simulink subsystem "PvtSubSys_VSM_ALL"  (R2020b)
settings: Solver=VariableStepAuto  StartTime=0.0  StopTime=10.0  RelTol=1e-3
values from neighbouring files (symbols this model uses):
  P_VSM_NOH_Act_Req = 0    [VSM_All.sldd]
  P_VSM_NOH_Swt_Req = 0    [VSM_All.sldd]
undefined symbols (not defined in the file or in its folder): ACC_STATE, HWA_STATE, LCK_STATE, P_VSM_ACCSOS_SW, P_VSM_AESSwtReq, P_VSM_CruiseFunUserInputMappingWays, P_VSM_ELKSwtReq, P_VSM_ESS_VehSwtReq, P_VSM_HWA_DMS_Enable, P_VSM_ICA_HandsOffSwtReq, P_VSM_IntelligentEvaSwtReq, P_VSM_ISLSwtReq, P_VSM_LCKSwtReq, P_VSM_LDWSwtReq, P_VSM_LKASwtReq, P_VSM_LSSSwtReq, P_VSM_PowerTrainConfig, P_VSM_SOSContinueTime, P_VSM_SOSSpdLimit, P_VSM_TSR_Dis_keep_SPL_Table, P_VSM_TSR_Dis_keep_SPLend, P_VSM_TSR_Dis_keep_TS_Table, P_VSM_TSR_Ena_SPLSupp_Table, P_VSM_TSR_Ena_TS_Table, P_VSM_TSR_SLIF_Speed_High, P_VSM_TSR_SLIF_Speed_Low, P_VSM_TSR_SLW_SnvtySwitch, P_VSM_TSR_SLW_Speed_Delta_disable, P_VSM_TSR_SLW_Speed_Delta_enable, P_VSM_TSR_SLW_Speed_High, P_VSM_TSR_SLW_Speed_Low, P_VSM_TSR_SLW_TrafEyeAvtiveDist, P_VSM_TSR_SLW_Warning_Time, P_VSM_TSR_SteerWheelAngle, P_VSM_TSR_SWS_speed_withDir, P_VSM_TSR_SWS_speed_woDir, P_VSM_TSRSwtReq, P_VSM_TSRWarnSwtReq, TJA_STATE, User_LC_ALCswt, User_LC_DrvConfirm, User_LC_DrvLCswt, User_LC_DrvOverride, User_LC_LeTurnNextLineReq, User_LC_RiTurnNextLineReq, User_LC_TurnMostLeLineReq, User_LC_TurnMostRiLineReq, User_LeTurnLmpOn, User_RiTurnLmpOn
libraries: simulink x51
(part 5 of 7)

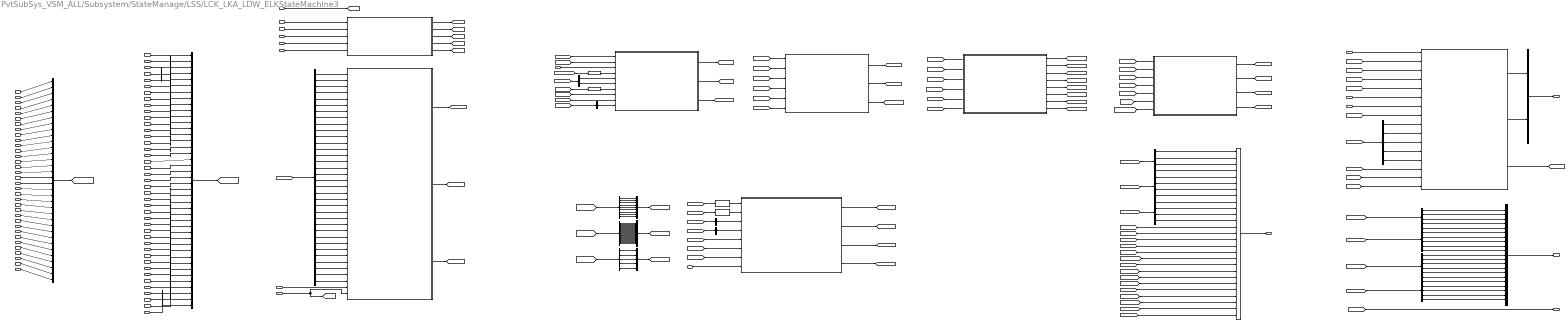
== system PvtSubSys_VSM_ALL/Subsystem/StateManage/LSS/LCK_LKA_LDW_ELKStateMachine3 ==
  VehConfig : Inport
  IFC_FailSafe : Inport  Port=2
  LCKError : Inport  Port=3
  LKAError : Inport  Port=4
  LDWError : Inport  Port=5
  ELKError : Inport  Port=6
  LCKLane_A0 : Inport  Port=7
  LCKLane_A1 : Inport  Port=8
  LCKLane_A2 : Inport  Port=9
  LCKLane_A3 : Inport  Port=10
  LCKLane_Valid : Inport  Port=11
  laneLeftA0 : Inport  Port=12
  laneLeftA1 : Inport  Port=13
  laneLeftA2 : Inport  Port=14
  laneLeftA3 : Inport  Port=15
  laneLeftValid : Inport  Port=16
  laneLeftRange : Inport  Port=17
  laneLeftType : Inport  Port=18
  laneRightA0 : Inport  Port=19
  laneRightA1 : Inport  Port=20
  laneRightA2 : Inport  Port=21
  laneRightA3 : Inport  Port=22
  laneRightValid : Inport  Port=23
  laneRightRange : Inport  Port=24
  laneRightType : Inport  Port=25
  F_LBbIsLineExist : Inport  Port=26
  F_LBdC0V : Inport  Port=27
  F_LBdC1V : Inport  Port=28
  F_LBdC2V : Inport  Port=29
  F_LBdC3V : Inport  Port=30
  RELeft_Range : Inport  Port=31
  F_RBbIsLineExist : Inport  Port=32
  F_RBdC0V : Inport  Port=33
  F_RBdC1V : Inport  Port=34
  F_RBdC2V : Inport  Port=35
  F_RBdC3V : Inport  Port=36
  RERight_Range : Inport  Port=37
  EVI_VehicleSpd_ms : Inport  Port=38
  EVI_Kap : Inport  Port=39
  EVI_alpSideSlipAngle : Inport  Port=40
  LCKIEBus : Inport  Port=41
  ELK_ObjBus : Inport  Port=42
  LIneEdgeUpdate : Inport  Port=43
  TrqK1 : Inport  Port=44
  targetExistP0 : Inport  Port=45
  HWALineValid : Inport  Port=46
  TJALineValid : Inport  Port=47
  LCKLineValid : Inport  Port=48
  HWAActive : Inport  Port=49
  TJASts : Inport  Port=50
  TJAOn : Inport  Port=51
  HWASts : Inport  Port=52
  canABSVehicleSpd : Inport  Port=53
  canABMVehDynYawRate : Inport  Port=54
  canESPVDCActive : Inport  Port=55
  canESPPTCActive : Inport  Port=56
  canESPBTCActive : Inport  Port=57
  canABSABSActive : Inport  Port=58
  HandsOffDetect : Inport  Port=59
  canSASSteerWheelAngle : Inport  Port=60
  canEPS_DriverInputTrqValue : Inport  Port=61
  canSASSteerWheelSpd : Inport  Port=62
  canABMLateralAcce : Inport  Port=63
  LongitudeAcc : Inport  Port=64
  canESP_MasterCylindBrakePress : Inport  Port=65
  canECMAccrPedlPosnDiagc : Inport  Port=66
  canEPS_LKATrqOvlDlvdSts : Inport  Port=67
  CURRENT_GEAR : Inport  Port=68
  canBCMLeftTurnSWSts : Inport  Port=69
  canBCMRightTurnSWSts : Inport  Port=70
  HandsOffWarnLevel : Inport  Port=71
  canBCMWiperSwitchSts : Inport  Port=72
  canBCMHighBeamSts : Inport  Port=73
  canBCMLowBeamSts : Inport  Port=74
  canBCMRearFogLmpSts : Inport  Port=75
  canBCMFrontFogLmpSts : Inport  Port=76
  canHUTLCKSwtReq : Inport  Port=77
  canHUTLKASwtReq : Inport  Port=78
  canHUTELKSwtReq : Inport  Port=79
  canHUTLDWSwtReq : Inport  Port=80
  IntelligentEvaSwtReq : Inport  Port=81
  IFC_SnvtySet : Inport  Port=82
  LSSSwtReq : Inport  Port=83
  ESSSts : Inport  Port=84
  PilotSts : Inport  Port=85
  BrkPedalSts : Inport  Port=86
  Bus Creator : BusCreator  Inputs=34
  Bus Creator1 : BusCreator  Inputs=27
  Bus Creator2 : BusCreator  Inputs=42
  Bus Creator3 : BusCreator  Inputs=9
  Bus Creator4 : BusCreator  Inputs=23
  Bus Creator5 : BusCreator  Inputs=5
  Bus Creator6 : BusCreator  Inputs=21
  Bus Selector : BusSelector  OutputSignals=LDW_Idle2Ready,LDW_Ready2Active,LDW_Active2Ready,LDW_Other2Idle
  Bus Selector11 : BusSelector  OutputSignals=Left_Valid,Right_Valid,Left_A0,Right_A0,C_Lanewidth
  Bus Selector12 : BusSelector  OutputSignals=LCKLane_A0,LCKLane_A1,LCKLane_A2,LCKLane_A3,LCKLane_Valid,laneLeftA0,laneLeftA1,laneLeftA2,laneLeftA3,laneLeftValid,laneLeftRange,laneLeftType,laneRightA0,laneRightA1,laneRightA2,laneRightA3,laneRightValid,laneRightRange,laneRightType,F_LBbIsLineExist,F_LBdC0V,F_LBdC1V,F_LBdC2V,F_LBdC3V,RELeft_Range,F_RBbIsLineExist,F_RBdC0V,F_RBdC1V,F_RBdC2V,F_RBdC3V,RERight_Range,EVI_VehicleSpd_ms,EVI_Kap,EVI_alpSideSlipAngle
  Bus Selector13 : BusSelector  OutputSignals=FLWhelDy,FRWhelDy
  Bus Selector14 : BusSelector  OutputSignals=Left_A0,Left_A1,Left_A2,Left_A3,Left_Valid,Right_A0,Right_A1,Right_A2,Right_A3,Right_Valid,LeftRE_A0,LeftRE_A1,LeftRE_A2,LeftRE_A3,LeftRE_Valid,RightRE_A0,RightRE_A1,RightRE_A2,RightRE_A3,RightRE_Valid,LaneCurve,LeftChange,RightChange
  Bus Selector15 : BusSelector  OutputSignals=LCK_Con_SteerAngleSpd_ LCKExit,LCK_Con_BrakePress_ LCKExit,LCK_Con_OverRide_ LCKExit,LCK_Con_AccPedalRate_LCKExit,LCK_Con_SteerWheelAngle_ LCKExit,LCK_Con_DriverInput_ LCKExit
  Bus Selector16 : BusSelector  OutputSignals=LKA_Con_SteerWheelAngle_ LKAExit,LKA_Con_DriverInput_ LKAExit,LKA_Con_SteerWheelSpd_ LKAExit,LKA_Con_BrakePressure_ LKAExit,LKA_Con_AccPedalRate_LKAExit,LKA_Con_OverRide_ LKAExit
  Bus Selector17 : BusSelector  OutputSignals=LDW_Con_AccPedalRate_LDWExit,LDW_Con_BrakePressure_ LDWExit,LDW_Con_SteerWheelSpd_ LDWExit,LDW_Con_SteerWheelAngle_ LDWExit,LDW_Con_DriverInput_ LDWExit
  Bus Selector2 : BusSelector  OutputSignals=VehConfigELK
  Bus Selector3 : BusSelector  OutputSignals=VehConfigLCKIE
  Bus Selector4 : BusSelector  OutputSignals=LKA_Idle2Ready,LKA_Ready2Active,LKA_Active2Ready,LKA_Other2Idle
  Bus Selector5 : BusSelector  OutputSignals=LCKLane_A0,LCKLane_A1,LCKLane_A2,LCKLane_A3,LCKLane_Valid
  Bus Selector6 : BusSelector  OutputSignals=IntelligentEvaSwtReq,canABSVehicleSpd,canBCMWiperSwitchSts,canBCMHighBeamSts,canBCMLowBeamSts,canBCMRearFogLmpSts,canBCMFrontFogLmpSts,canEPS_DriverInputTrqValue,HWASts
  Bus Selector7 : BusSelector  OutputSignals=EVI_VehicleSpd_ms
  Bus Selector8 : BusSelector  OutputSignals=VSM_ELK_Idle2Ready,VSM_ELK_Ready2Active,VSM_ELK_Active2Ready,VSM_ELK_Other2Idle
  Bus Selector9 : BusSelector  OutputSignals=ELK_Con_AccPedalRate_ELKExit,ELK_Con_BrakePressure_ ELKExit,ELK_Con_SteerWheelAngle_ ELKExit,ELK_Con_SteerWheelSpd_ ELKExit
  Bus Creator22 : BusCreator  Inputs=2
  Data Type Conversion : DataTypeConversion  OutDataTypeStr=boolean
  Data Type Conversion1 : DataTypeConversion  OutDataTypeStr=uint8
  Data Type Conversion2 : DataTypeConversion  OutDataTypeStr=boolean
  Data Type Conversion3 : DataTypeConversion  OutDataTypeStr=uint8
  ELKState_Machine : Subsystem
  Error : Subsystem
  HandsOffWarnLevel1 : InportShadow  Port=71
  LCK : Subsystem
  LCKIE : Subsystem  ReferencedSubsystem=PvtSubSys_VSM_LCKIE
  LDW : Subsystem
  LKA : Subsystem
  LSSHMI : Subsystem
  Signal_calculate : Subsystem  ReferencedSubsystem=PvtSubSys_VSM_SCM
  TJASts1 : InportShadow  Port=50
  canHUTLCKSwtReq1 : InportShadow  Port=77
  LCS_OutPut : Outport
  IFC_Signal : Outport  Port=2
  LSS_DATA : Outport  Port=3
  LaneARe_SP : Outport  Port=4
  wires:
  BrkPedalSts/1 -> Bus Creator2/42
  Bus Selector14/23 -> Bus Creator4/23  "<RightChange>"
  Bus Selector14/22 -> Bus Creator4/22  "<LeftChange>"
  [LANE] -> LCK/7(Lane)
  [PiloSts] -> LCK/6(PiloSts)
  PilotSts/1 -> Signal_calculate/36, [PiloSts]
  [TJA_LCKState] -> Bus Creator1/27  "TJA_LCKState"
  LCK/4(TJA_LCKState) -> [TJA_LCKState]
  [LaneARe_SP] -> LaneARe_SP/1
  Data Type Conversion3/1 -> ELKState_Machine/4(LKAState)
  Bus Creator6/1 -> LSS_DATA/1
  Bus Selector17/5 -> Bus Creator6/21  "<LDW_Con_DriverInput_ LDWExit>"
  Bus Selector17/4 -> Bus Creator6/20  "<LDW_Con_SteerWheelAngle_ LDWExit>"
  Bus Selector17/3 -> Bus Creator6/19  "<LDW_Con_SteerWheelSpd_ LDWExit>"
  Bus Selector17/2 -> Bus Creator6/18  "<LDW_Con_BrakePressure_ LDWExit>"
  Bus Selector17/1 -> Bus Creator6/17  "<LDW_Con_AccPedalRate_LDWExit>"
  Bus Selector16/6 -> Bus Creator6/16  "<LKA_Con_OverRide_ LKAExit>"
  Bus Selector15/1 -> Bus Creator6/5  "<LCK_Con_SteerAngleSpd_ LCKExit>"
  Bus Selector16/5 -> Bus Creator6/15  "<LKA_Con_AccPedalRate_LKAExit>"
  Bus Selector15/2 -> Bus Creator6/6  "<LCK_Con_BrakePress_ LCKExit>"
  Bus Selector16/4 -> Bus Creator6/14  "<LKA_Con_BrakePressure_ LKAExit>"
  Bus Selector15/3 -> Bus Creator6/7  "<LCK_Con_OverRide_ LCKExit>"
  Bus Selector9/4 -> Bus Creator6/4  "<ELK_Con_SteerWheelSpd_ ELKExit>"
  Bus Selector16/3 -> Bus Creator6/13  "<LKA_Con_SteerWheelSpd_ LKAExit>"
  Bus Selector16/1 -> Bus Creator6/11  "<LKA_Con_SteerWheelAngle_ LKAExit>"
  Bus Selector15/6 -> Bus Creator6/10  "<LCK_Con_DriverInput_ LCKExit>"
  Bus Selector15/4 -> Bus Creator6/8  "<LCK_Con_AccPedalRate_LCKExit>"
  Bus Selector9/3 -> Bus Creator6/3  "<ELK_Con_SteerWheelAngle_ ELKExit>"
  Bus Selector9/1 -> Bus Creator6/1  "<ELK_Con_AccPedalRate_ELKExit>"
  Bus Selector16/2 -> Bus Creator6/12  "<LKA_Con_DriverInput_ LKAExit>"
  Bus Selector15/5 -> Bus Creator6/9  "<LCK_Con_SteerWheelAngle_ LCKExit>"
  Bus Selector9/2 -> Bus Creator6/2  "<ELK_Con_BrakePressure_ ELKExit>"
  [LDW_Data] -> Bus Selector17/1
  [LKA_Data] -> Bus Selector16/1
  [LCK_Data] -> Bus Selector15/1
  [ELKCondition] -> Bus Selector9/1
  LSSHMI/3(Warn) -> [LKAWarning]
  LSSHMI/2(LaneAvaliability) -> Bus Creator22/2
  LSSHMI/1(Signal_HandsOffWarn) -> Bus Creator22/1
  TJASts1/1 -> LSSHMI/7(TJASts)  "TJASts"
  HandsOffWarnLevel1/1 -> LSSHMI/6(HandsOffWarnLevel)  "HandsOffWarnLevel"
  [LCK_State] -> LSSHMI/8(In8)
  [LKA_State] -> LSSHMI/5(In5)
  [ELK_State] -> LSSHMI/4(In4)
  [ELKWarn] -> LSSHMI/16(ELK_Warn)
  [LKA_Warn] -> LSSHMI/15(In15)
  [LCK_Warn] -> LSSHMI/14(LCK_Warn)
  Bus Selector11/5 -> LSSHMI/13(LaneWidth)  "<C_Lanewidth>"
  Bus Selector11/4 -> LSSHMI/12(RightA0)  "<Right_A0>"
  Bus Selector11/3 -> LSSHMI/11(LeftA0)  "<Left_A0>"
  Bus Selector11/1 -> LSSHMI/9(LeftValid)  "<Left_Valid>"
  Bus Selector11/2 -> LSSHMI/10(RightValid)  "<Right_Valid>"
  [LDW_State] -> LSSHMI/3(In3)
  [LCK_State] -> LSSHMI/2(In2)
  canHUTLCKSwtReq1/1 -> LSSHMI/1(canHUTLCKSwtReq)  "canHUTLCKSwtReq"
  [VSM_LCKIE_out] -> Bus Creator1/26
  [VSM_LCKIE_IN] -> Bus Creator1/25
  LCKIE/4 -> [VSM_LCKIE_out]
  LCKIE/3 -> [VSM_LCKIE_IN]
  Bus Selector13/2 -> ELKState_Machine/6(FRWhelDy)  "<FRWhelDy>"
  Bus Selector13/1 -> ELKState_Machine/5(FLWhelDy)  "<FLWhelDy>"
  [LKA_LDW_Signal] -> Bus Selector13/1
  [ADmix] -> LDW/5(ADmix)
  [VehConfig] -> LKA/4(VehConfig)
  [LaneARe_SP] -> LDW/4(LaneARe_SP)
  [VehConfig] -> LDW/1(VehConfig)
  LCK/2(LCK_Warn) -> [LCK_Warn]
  [LDW_Error] -> LDW/2(LDW_Error)
  LKA/2(LKA_State) -> [LKA_State]
  [LKA_LDW_Signal] -> LDW/3(LKA_LDW_Signal)
  LKA/8(LKACondition) -> [LKACondition]
  [LKA_LDW_Signal] -> LKA/2(LKA_LDW_Signal)
  LDW/1(LDW_State) -> [LDW_State]
  LDW/2(LDWData) -> [LDW_Data]
  [LaneARe_SP] -> LKA/1(LaneARe_SP)
  [FailSafe] -> LKA/6(FailSafe)
  LKA/3(LKADesLaneDyoffset_m) -> [LKADesLaneDyoffset_m]
  [ADmix] -> LKA/5(ADmix)
  LCK/3(LCK_State) -> [LCK_State]
  LKA/7(LKA_InterventionEnd) -> [LKA_InterventionEnd]
  LKA/1(LKAData) -> [LKA_Data]
  LKA/5(LKA_LKAactive) -> [LKA_LKAactive]
  LKA/6(LKA_LKAout) -> [LKA_LKAout]
  [LKA_LDW_Signal] -> LCK/3(LKA_LDW_Signal)
  [LaneARe_SP] -> LCK/5(LaneARe_SP)
  [ADmix] -> LCK/4(ADmix)
  [FailSafe] -> LDW/6(FailSafe)
  [LKA_Error] -> LKA/3(LKA_Error)
  LKA/4(LKA_Warn) -> [LKA_Warn]
  [LCK_Error] -> LCK/1(LCK_Error)
  LDW/3(LDWCondition) -> [LDWCondition]
  [VehConfig] -> LCK/2(VehConfig)
  LCK/1(LCKData) -> [LCK_Data]
  Data Type Conversion2/1 -> LCKIE/2
  LCKIE/2 -> [LCKIE_Laneoffset]
  LCKIE/1 -> [LCKIE_State]
  [LCKIE_CenterLane] -> LCKIE/7
  [LCKIE_LANE] -> LCKIE/6
  [LCKIE_ADCAN] -> LCKIE/5
  Bus Selector7/1 -> LCKIE/4  "<EVI_VehicleSpd_ms>"
  Bus Selector3/1 -> LCKIE/3  "<VehConfigLCKIE>"
  [FailSafe] -> Data Type Conversion2/1
  Data Type Conversion1/1 -> LCKIE/1
  [LANE] -> Bus Selector7/1
  [VehConfig] -> Bus Selector3/1
  [LCK_State] -> Data Type Conversion1/1
  Bus Selector6/2 -> Bus Creator3/2  "<canABSVehicleSpd>"
  Bus Selector6/8 -> Bus Creator3/8  "<canEPS_DriverInputTrqValue>"
  Bus Selector14/4 -> Bus Creator4/4  "<Left_A3>"
  Bus Selector6/6 -> Bus Creator3/6  "<canBCMRearFogLmpSts>"
  Bus Selector6/3 -> Bus Creator3/3  "<canBCMWiperSwitchSts>"
  Bus Selector5/3 -> Bus Creator5/3  "<LCKLane_A2>"
  Bus Creator4/1 -> [LCKIE_LANE]
  Bus Selector14/5 -> Bus Creator4/5  "<Left_Valid>"
  [ADmix] -> Bus Selector6/1
  Bus Selector6/9 -> Bus Creator3/9  "<HWASts>"
  Bus Selector14/6 -> Bus Creator4/6  "<Right_A0>"
  Bus Selector6/5 -> Bus Creator3/5  "<canBCMLowBeamSts>"
  Bus Selector6/7 -> Bus Creator3/7  "<canBCMFrontFogLmpSts>"
  Bus Selector14/3 -> Bus Creator4/3  "<Left_A2>"
  Bus Selector14/12 -> Bus Creator4/12  "<LeftRE_A1>"
  Bus Selector14/9 -> Bus Creator4/9  "<Right_A3>"
  Bus Selector14/8 -> Bus Creator4/8  "<Right_A2>"
  Bus Selector14/15 -> Bus Creator4/15  "<LeftRE_Valid>"
  Bus Selector14/19 -> Bus Creator4/19  "<RightRE_A3>"
  Bus Selector14/16 -> Bus Creator4/16  "<RightRE_A0>"
  Bus Selector14/7 -> Bus Creator4/7  "<Right_A1>"
  Bus Selector14/11 -> Bus Creator4/11  "<LeftRE_A0>"
  Bus Selector14/1 -> Bus Creator4/1  "<Left_A0>"
  Bus Selector14/21 -> Bus Creator4/21  "<LaneCurve>"
  Bus Selector14/14 -> Bus Creator4/14  "<LeftRE_A3>"
  Bus Creator5/1 -> [LCKIE_CenterLane]
  Bus Selector14/18 -> Bus Creator4/18  "<RightRE_A2>"
  Bus Selector5/1 -> Bus Creator5/1  "<LCKLane_A0>"
  Bus Selector5/4 -> Bus Creator5/4  "<LCKLane_A3>"
  Bus Selector14/13 -> Bus Creator4/13  "<LeftRE_A2>"
  Bus Selector5/2 -> Bus Creator5/2  "<LCKLane_A1>"
  Bus Selector14/17 -> Bus Creator4/17  "<RightRE_A1>"
  [LANE] -> Bus Selector5/1
  Bus Creator3/1 -> [LCKIE_ADCAN]
  Bus Selector14/2 -> Bus Creator4/2  "<Left_A1>"
  Bus Selector14/10 -> Bus Creator4/10  "<Right_Valid>"
  Bus Selector14/20 -> Bus Creator4/20  "<RightRE_Valid>"
  Bus Selector6/4 -> Bus Creator3/4  "<canBCMHighBeamSts>"
  Bus Selector5/5 -> Bus Creator5/5  "<LCKLane_Valid>"
  Bus Selector6/1 -> Bus Creator3/1  "<IntelligentEvaSwtReq>"
  [LaneARe_SP] -> Bus Selector14/1
  Data Type Conversion/1 -> ELKState_Machine/7(IFC_Failsafe)
  [LKA_State] -> Data Type Conversion3/1
  Bus Creator22/1 -> IFC_Signal/1
  VehConfig/1 -> [VehConfig]
  Signal_calculate/2 -> [LaneARe_SP]  "LaneARe_SP"
  IFC_FailSafe/1 -> Error/1(IFC_FailSafe)
  LCKError/1 -> Error/2(LCKError)
  ELKError/1 -> Error/5(ELKError)
  LDWError/1 -> Error/4(LDWError)
  LKAError/1 -> Error/3(LKAError)
  Error/1(FailSafe) -> [FailSafe]
  Error/2(LCK_Error) -> [LCK_Error]
  Error/3(LKA_Error) -> [LKA_Error]
  Error/4(LDW_Error) -> [LDW_Error]
  Error/5(ELK_Error) -> [ELK_Error]
  Signal_calculate/3 -> [LKA_LDW_Signal]
  Signal_calculate/1 -> [Lane_Re]
  [LDWCondition] -> Bus Selector/1
  [LKACondition] -> Bus Selector4/1
  [ELKCondition] -> Bus Selector8/1
  Bus Selector/1 -> Bus Creator1/1  "<LDW_Idle2Ready>"
  Bus Selector/2 -> Bus Creator1/2  "<LDW_Ready2Active>"
  Bus Selector/3 -> Bus Creator1/3  "<LDW_Active2Ready>"
  Bus Selector/4 -> Bus Creator1/4  "<LDW_Other2Idle>"
  Bus Selector4/1 -> Bus Creator1/5  "<LKA_Idle2Ready>"
  Bus Selector4/2 -> Bus Creator1/6  "<LKA_Ready2Active>"
  Bus Selector4/3 -> Bus Creator1/7  "<LKA_Active2Ready>"
  Bus Selector4/4 -> Bus Creator1/8  "<LKA_Other2Idle>"
  Bus Creator1/1 -> LCS_OutPut/1
  [LCK_State] -> Bus Creator1/13  "LCK_State"
  [LKA_State] -> Bus Creator1/14  "LKA_State"
  [LDW_State] -> Bus Creator1/15  "LDW_State"
  [LCKIE_State] -> Bus Creator1/16  "LCKIE_State"
  [ELK_State] -> Bus Creator1/17  "ELK_State"
  [LKA_LKAactive] -> Bus Creator1/21  "LKA_LKAactive"
  [LKA_LKAout] -> Bus Creator1/22  "LKA_LKAout"
  [LKADesLaneDyoffset_m] -> Bus Creator1/18  "LKADesLaneDyoffset_m"
  [LKA_InterventionEnd] -> Bus Creator1/20  "LKA_InterventionEnd"
  [LDW_warnflag] -> Bus Creator1/24  "LDW_warnflag"
  [LKAWarning] -> Bus Creator1/19  "LKAWarning"
  [LCKIE_Laneoffset] -> Bus Creator1/23  "LCKIE_Laneoffset"
  [LaneARe_SP] -> Bus Selector11/1
  IFC_SnvtySet/1 -> Bus Creator2/41  "IFC_SnvtySet"
  LCKLane_A0/1 -> Bus Creator/1  "LCKLane_A0"
  LCKLane_A1/1 -> Bus Creator/2  "LCKLane_A1"
  LCKLane_A2/1 -> Bus Creator/3  "LCKLane_A2"
  LCKLane_A3/1 -> Bus Creator/4  "LCKLane_A3"
  LCKLane_Valid/1 -> Bus Creator/5  "LCKLane_Valid"
  laneLeftA0/1 -> Bus Creator/6  "laneLeftA0"
  laneLeftA1/1 -> Bus Creator/7  "laneLeftA1"
  laneLeftA2/1 -> Bus Creator/8  "laneLeftA2"
  laneLeftA3/1 -> Bus Creator/9  "laneLeftA3"
  laneLeftValid/1 -> Bus Creator/10  "laneLeftValid"
  laneLeftRange/1 -> Bus Creator/11  "laneLeftRange"
  laneLeftType/1 -> Bus Creator/12  "laneLeftType"
  laneRightA0/1 -> Bus Creator/13  "laneRightA0"
  laneRightA1/1 -> Bus Creator/14  "laneRightA1"
  laneRightA2/1 -> Bus Creator/15  "laneRightA2"
  laneRightA3/1 -> Bus Creator/16  "laneRightA3"
  laneRightValid/1 -> Bus Creator/17  "laneRightValid"
  laneRightRange/1 -> Bus Creator/18  "laneRightRange"
  laneRightType/1 -> Bus Creator/19  "laneRightType"
  F_LBbIsLineExist/1 -> Bus Creator/20  "F_LBbIsLineExist"
  F_LBdC0V/1 -> Bus Creator/21  "F_LBdC0V"
  F_LBdC1V/1 -> Bus Creator/22  "F_LBdC1V"
  F_LBdC2V/1 -> Bus Creator/23  "F_LBdC2V"
  F_LBdC3V/1 -> Bus Creator/24  "F_LBdC3V"
  RELeft_Range/1 -> Bus Creator/25  "RELeft_Range"
  F_RBbIsLineExist/1 -> Bus Creator/26  "F_RBbIsLineExist"
  F_RBdC0V/1 -> Bus Creator/27  "F_RBdC0V"
  F_RBdC1V/1 -> Bus Creator/28  "F_RBdC1V"
  F_RBdC2V/1 -> Bus Creator/29  "F_RBdC2V"
  F_RBdC3V/1 -> Bus Creator/30  "F_RBdC3V"
  RERight_Range/1 -> Bus Creator/31  "RERight_Range"
  EVI_VehicleSpd_ms/1 -> Bus Creator/32  "EVI_VehicleSpd_ms"
  EVI_Kap/1 -> Bus Creator/33  "EVI_Kap"
  EVI_alpSideSlipAngle/1 -> Bus Creator/34  "EVI_alpSideSlipAngle"
  LCKIEBus/1 -> LCKIE/8  "LCKIEBus"
  ELK_ObjBus/1 -> ELKState_Machine/3(TOS_ELK)  "ELK_ObjBus"
  LIneEdgeUpdate/1 -> Signal_calculate/35  "LIneEdgeUpdate"
  Bus Creator/1 -> [LANE]
  TJASts/1 -> Bus Creator2/7  "TJASts"
  LCKLineValid/1 -> Bus Creator2/6  "LCKLineValid"
  TJAOn/1 -> Bus Creator2/8  "TJAOn"
  TJALineValid/1 -> Bus Creator2/5  "TJALineValid"
  HWASts/1 -> Bus Creator2/9  "HWASts"
  HWAActive/1 -> Bus Creator2/4  "HWAActive"
  HandsOffDetect/1 -> Bus Creator2/10
  HandsOffWarnLevel/1 -> Bus Creator2/11  "HandsOffWarnLevel"
  ESSSts/1 -> Bus Creator2/12  "ESSSts"
  HWALineValid/1 -> Bus Creator2/3  "HWALineValid"
  targetExistP0/1 -> Bus Creator2/2  "targetExistP0"
  canABSVehicleSpd/1 -> Bus Creator2/13  "canABSVehicleSpd"
  TrqK1/1 -> Bus Creator2/1  "TrqK1"
  canABMVehDynYawRate/1 -> Bus Creator2/14  "canABMVehDynYawRate"
  canESPVDCActive/1 -> Bus Creator2/15  "canESPVDCActive"
  canESPPTCActive/1 -> Bus Creator2/16  "canESPPTCActive"
  canESPBTCActive/1 -> Bus Creator2/17  "canESPBTCActive"
  canABSABSActive/1 -> Bus Creator2/18  "canABSABSActive"
  canSASSteerWheelAngle/1 -> Bus Creator2/19  "canSASSteerWheelAngle"
  canEPS_DriverInputTrqValue/1 -> Bus Creator2/20  "canEPS_DriverInputTrqValue"
  canSASSteerWheelSpd/1 -> Bus Creator2/21  "canSASSteerWheelSpd"
  canABMLateralAcce/1 -> Bus Creator2/22  "canABMLateralAcce"
  LongitudeAcc/1 -> Bus Creator2/23  "LongitudeAcc"
  canESP_MasterCylindBrakePress/1 -> Bus Creator2/24  "canESP_MasterCylindBrakePress"
  canECMAccrPedlPosnDiagc/1 -> Bus Creator2/25  "canECMAccrPedlPosnDiagc"
  canEPS_LKATrqOvlDlvdSts/1 -> Bus Creator2/26  "canEPS_LKATrqOvlDlvdSts"
  CURRENT_GEAR/1 -> Bus Creator2/27  "CURRENT_GEAR"
  canBCMLeftTurnSWSts/1 -> Bus Creator2/28  "canBCMLeftTurnSWSts"
  canBCMRightTurnSWSts/1 -> Bus Creator2/29  "canBCMRightTurnSWSts"
  canBCMWiperSwitchSts/1 -> Bus Creator2/30  "canBCMWiperSwitchSts"
  canBCMHighBeamSts/1 -> Bus Creator2/31  "canBCMHighBeamSts"
  canBCMLowBeamSts/1 -> Bus Creator2/32  "canBCMLowBeamSts"
  canBCMRearFogLmpSts/1 -> Bus Creator2/33  "canBCMRearFogLmpSts"
  canBCMFrontFogLmpSts/1 -> Bus Creator2/34  "canBCMFrontFogLmpSts"
  canHUTLCKSwtReq/1 -> Bus Creator2/35  "canHUTLCKSwtReq"
  Bus Creator2/1 -> [ADmix]
  [LANE] -> Bus Selector12/1
  Bus Selector12/1 -> Signal_calculate/1  "<LCKLane_A0>"
  Bus Selector12/2 -> Signal_calculate/2  "<LCKLane_A1>"
  Bus Selector12/3 -> Signal_calculate/3  "<LCKLane_A2>"
  Bus Selector12/4 -> Signal_calculate/4  "<LCKLane_A3>"
  Bus Selector12/5 -> Signal_calculate/5  "<LCKLane_Valid>"
  Bus Selector12/6 -> Signal_calculate/6  "<laneLeftA0>"
  Bus Selector12/7 -> Signal_calculate/7  "<laneLeftA1>"
  Bus Selector12/8 -> Signal_calculate/8  "<laneLeftA2>"
  Bus Selector12/9 -> Signal_calculate/9  "<laneLeftA3>"
  Bus Selector12/10 -> Signal_calculate/10  "<laneLeftValid>"
  Bus Selector12/11 -> Signal_calculate/11  "<laneLeftRange>"
  Bus Selector12/12 -> Signal_calculate/12  "<laneLeftType>"
  Bus Selector12/13 -> Signal_calculate/13  "<laneRightA0>"
  Bus Selector12/14 -> Signal_calculate/14  "<laneRightA1>"
  Bus Selector12/15 -> Signal_calculate/15  "<laneRightA2>"
  Bus Selector12/16 -> Signal_calculate/16  "<laneRightA3>"
  Bus Selector12/17 -> Signal_calculate/17  "<laneRightValid>"
  Bus Selector12/18 -> Signal_calculate/18  "<laneRightRange>"
  Bus Selector12/19 -> Signal_calculate/19  "<laneRightType>"
  Bus Selector12/20 -> Signal_calculate/20  "<F_LBbIsLineExist>"
  Bus Selector12/21 -> Signal_calculate/21  "<F_LBdC0V>"
  Bus Selector12/22 -> Signal_calculate/22  "<F_LBdC1V>"
  Bus Selector12/23 -> Signal_calculate/23  "<F_LBdC2V>"
  Bus Selector12/24 -> Signal_calculate/24  "<F_LBdC3V>"
  Bus Selector12/25 -> Signal_calculate/25  "<RELeft_Range>"
  Bus Selector12/26 -> Signal_calculate/26  "<F_RBbIsLineExist>"
  Bus Selector12/27 -> Signal_calculate/27  "<F_RBdC0V>"
  Bus Selector12/28 -> Signal_calculate/28  "<F_RBdC1V>"
  Bus Selector12/29 -> Signal_calculate/29  "<F_RBdC2V>"
  Bus Selector12/30 -> Signal_calculate/30  "<F_RBdC3V>"
  Bus Selector12/31 -> Signal_calculate/31  "<RERight_Range>"
  Bus Selector12/32 -> Signal_calculate/32  "<EVI_VehicleSpd_ms>"
  Bus Selector12/33 -> Signal_calculate/33  "<EVI_Kap>"
  Bus Selector12/34 -> Signal_calculate/34  "<EVI_alpSideSlipAngle>"
  [ADmix] -> ELKState_Machine/9(ADBUS)
  canHUTLKASwtReq/1 -> Bus Creator2/36  "canHUTLKASwtReq"
  canHUTELKSwtReq/1 -> Bus Creator2/37  "canHUTELKSwtReq"
  canHUTLDWSwtReq/1 -> Bus Creator2/38  "canHUTLDWSwtReq"
  IntelligentEvaSwtReq/1 -> Bus Creator2/39  "IntelligentEvaSwtReq"
  LSSSwtReq/1 -> Bus Creator2/40  "LSSSwtReq"
  [VehConfig] -> Bus Selector2/1
  Bus Selector2/1 -> ELKState_Machine/10(VehConfigELK)  "<VehConfigELK>"
  [LaneARe_SP] -> ELKState_Machine/1(LaneARe_SP)
  [LANE] -> ELKState_Machine/2(Lane)
  [ELK_Error] -> ELKState_Machine/8(canHUTELKError)
  [FailSafe] -> Data Type Conversion/1
  ELKState_Machine/1(ELKstate) -> [ELK_State]
  ELKState_Machine/2(warn) -> [ELKWarn]
  ELKState_Machine/3(ELK_Data) -> [ELKCondition]
  Bus Selector8/1 -> Bus Creator1/9  "<VSM_ELK_Idle2Ready>"
  Bus Selector8/2 -> Bus Creator1/10  "<VSM_ELK_Ready2Active>"
  Bus Selector8/3 -> Bus Creator1/11  "<VSM_ELK_Active2Ready>"
  Bus Selector8/4 -> Bus Creator1/12  "<VSM_ELK_Other2Idle>"

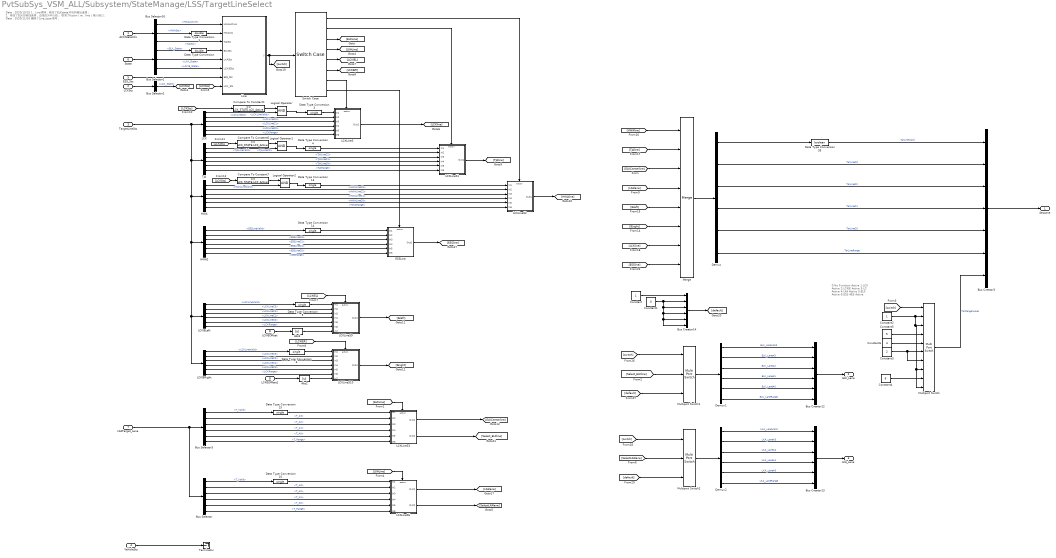
== system PvtSubSys_VSM_ALL/Subsystem/StateManage/LSS/TargetLineSelect ==
  note: 0:No Function Active
      | 1:LCK Active
      | 2:LCKIE Active
      | 3:LC Active
      | 4:LKA Active
      | 5:ELK Active
      | 6:ESS AES Active
  note: Data：2020/10/15
      | 1、Line模块：修改了ELKstate对应的输出选择；
      | 2、修改了ELK目标线选择，边线改为中心线；
      | 取消了fusion（re、line）输入接口；
      | Data：2020/11/03
      | 删除了Line_type信号；
  ACCStateInfo : Inport
  LCKSts : Inport  Port=2
  TargetLineSts : Inport  Port=3
  VehicleSts : Inport  Port=4
  "ESS_Sts " : Inport  Port=5
  "State " : Inport  Port=6
  "LKATarget_Lane " : Inport  Port=7
  LCKIEOffset : Inport  Port=8
  Abs2 : Abs
  Abs3 : Abs
  Bus Creator12 : BusCreator  Inputs=6
  Bus Creator13 : BusCreator  Inputs=6
  Bus Creator14 : BusCreator  Inputs=6
  Bus Selector : BusSelector  OutputSignals=T_Valid,T_A3,T_A2,T_A1,T_A0,T_Range
  Bus Selector3 : BusSelector  OutputSignals=T_Valid,T_A3,T_A2,T_A1,T_A0,T_Range
  Bus Creator3 : BusCreator  Inputs=7
  Bus Selector1 : BusSelector  OutputSignals=ELK_State,LKA_State,LCKIE_State
  Bus Selector16 : BusSelector  OutputSignals=HWAActive,HWASts,TJASts
  Bus Selector2 : BusSelector  OutputSignals=LCK_State
  Compare To Constant1 : simulink/Logic and Bit Operations/Compare To Constant  relop===  const=LCK_STATE.LCK_Active  OutDataTypeStr=boolean
  Compare To Constant6 : simulink/Logic and Bit Operations/Compare To Constant  relop===  const=LCK_STATE.LCK_Active  OutDataTypeStr=boolean
  Compare To Constant7 : simulink/Logic and Bit Operations/Compare To Constant  relop===  const=LCK_STATE.LCK_Active  OutDataTypeStr=boolean
  Constant : Constant
  Constant1 : Constant  Value=0
  Constant2 : Constant  OutDataTypeStr=uint8
  Constant3 : Constant  Value=2  OutDataTypeStr=uint8
  Constant4 : Constant  Value=6  OutDataTypeStr=uint8
  Constant5 : Constant  Value=5  OutDataTypeStr=uint8
  Constant6 : Constant  Value=4  OutDataTypeStr=uint8
  Data Type Conversion : DataTypeConversion  OutDataTypeStr=double
  Data Type Conversion1 : DataTypeConversion  OutDataTypeStr=double
  Data Type Conversion{3..6,10,13..15} (8 alike) : DataTypeConversion  OutDataTypeStr=single
  Data Type Conversion35 : DataTypeConversion  OutDataTypeStr=boolean
  Demux : Demux  Outputs=6
  Demux1 : Demux  Outputs=6
  Demux2 : Demux  Outputs=6
  ESSLine : Subsystem  TreatAsAtomicUnit=on
  HWA : BusSelector  OutputSignals=LSM_HWA.HWALineValid,LSM_HWA.HWALineC3,LSM_HWA.HWALineC2,LSM_HWA.HWALineC1,LSM_HWA.HWALineC0,LSM_HWA.HWARange
  HWA2 : BusSelector  OutputSignals=LSM_ESS.ESSLineValid,LSM_ESS.ESSLineC3,LSM_ESS.ESSLineC2,LSM_ESS.ESSLineC1,LSM_ESS.ESSLineC0,LSM_ESS.ESSRange
  LCK : BusSelector  OutputSignals=LSM_LCK.LCKLineValid,LSM_LCK.LCKLineC3,LSM_LCK.LCKLineC2,LSM_LCK.LCKLineC1,LSM_LCK.LCKLineC0,LSM_LCK.LCKRange
  LCKIELeft : BusSelector  OutputSignals=LSM_LCK.LCKLineValid,LSM_LCK.LCKLineC3,LSM_LCK.LCKLineC2,LSM_LCK.LCKLineC1,LSM_LCK.LCKLineC0,LSM_LCK.LCKRange
  LCKIEOffset1 : InportShadow  Port=8
  LCKIERight : BusSelector  OutputSignals=LSM_LCK.LCKLineValid,LSM_LCK.LCKLineC3,LSM_LCK.LCKLineC2,LSM_LCK.LCKLineC1,LSM_LCK.LCKLineC0,LSM_LCK.LCKRange
  LCKLineS : Subsystem  TreatAsAtomicUnit=on
  LCKLineS1 : Subsystem  TreatAsAtomicUnit=on
  LCKLineS10 : Subsystem  TreatAsAtomicUnit=on
  LCKLineS2 : Subsystem  TreatAsAtomicUnit=on
  LCKLineS3 : Subsystem  TreatAsAtomicUnit=on
  LCKLineS6 : Subsystem  TreatAsAtomicUnit=on
  LCKLineS9 : Subsystem  TreatAsAtomicUnit=on
  Line : MATLAB Function  TreatAsAtomicUnit=on
  Logical Operator : Logic  AllPortsSameDT=off  OutDataTypeStr=boolean
  Logical Operator1 : Logic  AllPortsSameDT=off  OutDataTypeStr=boolean
  Logical Operator2 : Logic  AllPortsSameDT=off  OutDataTypeStr=boolean
  Merge : Merge  Inputs=8
  Multiport Switch : MultiPortSwitch  Inputs=9
  Multiport Switch1 : MultiPortSwitch  DataPortOrder=Specify indices  Inputs=4  DataPortIndices={3,7}  DiagnosticForDefault=None
  Multiport Switch2 : MultiPortSwitch  DataPortOrder=Specify indices  Inputs=4  DataPortIndices={7,8}  DiagnosticForDefault=None
  Switch Case : SwitchCase  CaseConditions={1,2,3,4,5,6,7,8}  ShowDefaultCase=off
  TJA : BusSelector  OutputSignals=LSM_TJA_ICA.TJALineValid,LSM_TJA_ICA.TJALineC3,LSM_TJA_ICA.TJALineC2,LSM_TJA_ICA.TJALineC1,LSM_TJA_ICA.TJALineC0,LSM_TJA_ICA.TJARange
  Terminator : Terminator
  desLane : Outport
  ELK_Lane : Outport  Port=2
  LKA_Lane : Outport  Port=3
  wires:
  [LCKSts] -> Compare To Constant7/1
  [LCKSts] -> Compare To Constant6/1
  [LCKSts] -> Compare To Constant1/1
  [LCKSts] -> Line/8(LCK_Sts)
  Constant6/1 -> Multiport Switch/5
  Constant5/1 -> Multiport Switch/4
  Constant4/1 -> Multiport Switch/9
  Constant3/1 -> Multiport Switch/6, Multiport Switch/7
  Constant2/1 -> Multiport Switch/2, Multiport Switch/3, Multiport Switch/8, Multiport Switch/10
  [switch] -> Multiport Switch/1
  Multiport Switch/1 -> Bus Creator3/7  "TarDangerLevel"
  Data Type Conversion15/1 -> LCKLineS3/1(In1)
  [ESSline] -> Merge/8
  [LCKline] -> Merge/7
  [IEright] -> Merge/6
  [IEleft] -> Merge/5
  [LKAlane] -> Merge/4
  Switch Case/6 -> [LCKIER]
  Switch Case/5 -> [LCKIEL]
  Switch Case/4 -> [LKALine]
  Bus Selector3/6 -> LCKLineS3/6(In6)  "<T_Range>"
  Bus Selector3/5 -> LCKLineS3/5(In5)  "<T_A0>"
  Bus Selector3/4 -> LCKLineS3/4(In4)  "<T_A1>"
  Bus Selector3/3 -> LCKLineS3/3(In3)  "<T_A2>"
  Bus Selector3/2 -> LCKLineS3/2(In2)  "<T_A3>"
  Bus Selector3/1 -> Data Type Conversion15/1  "<T_Valid>"
  "LKATarget_Lane "/1 -> Bus Selector/1, Bus Selector3/1
  Logical Operator2/1 -> Data Type Conversion13/1
  Compare To Constant7/1 -> Logical Operator2/1
  Logical Operator1/1 -> Data Type Conversion4/1
  Compare To Constant6/1 -> Logical Operator1/1
  Demux/6 -> Bus Creator3/6  "TarLineRange"
  Demux/5 -> Bus Creator3/5  "TarLineC0"
  Bus Selector16/3 -> Line/3(TJASts)  "<TJASts>"
  ACCStateInfo/1 -> Bus Selector16/1
  Bus Selector16/1 -> Line/1(HWAActive)  "<HWAActive>"
  Bus Creator3/1 -> desLane/1
  Demux/4 -> Bus Creator3/4  "TarLineC1"
  Switch Case/2 -> LCKLineS1/Action
  Switch Case/1 -> LCKLineS2/Action
  Demux/2 -> Bus Creator3/2  "TarLineC3"
  HWA/4 -> LCKLineS2/4(In4)  "<HWALineC1>"
  Demux/3 -> Bus Creator3/3  "TarLineC2"
  HWA/6 -> LCKLineS2/6(In6)  "<HWARange>"
  HWA/2 -> LCKLineS2/2(In2)  "<HWALineC3>"
  HWA/3 -> LCKLineS2/3(In3)  "<HWALineC2>"
  HWA/5 -> LCKLineS2/5(In5)  "<HWALineC0>"
  HWA/1 -> Logical Operator2/2  "<HWALineValid>"
  TJA/3 -> LCKLineS1/3(In3)  "<TJALineC2>"
  TJA/6 -> LCKLineS1/6(In6)  "<TJARange>"
  TJA/1 -> Logical Operator1/2  "<TJALineValid>"
  TJA/2 -> LCKLineS1/2(In2)  "<TJALineC3>"
  TJA/4 -> LCKLineS1/4(In4)  "<TJALineC1>"
  TJA/5 -> LCKLineS1/5(In5)  "<TJALineC0>"
  LCK/3 -> LCKLineS/3(In3)  "<LCKLineC2>"
  LCK/5 -> LCKLineS/5(In5)  "<LCKLineC0>"
  LCK/4 -> LCKLineS/4(In4)  "<LCKLineC1>"
  LCK/2 -> LCKLineS/2(In2)  "<LCKLineC3>"
  LCK/6 -> LCKLineS/6(In6)  "<LCKRange>"
  VehicleSts/1 -> Terminator/1
  TargetLineSts/1 -> LCK/1, TJA/1, HWA2/1, LCKIERight/1, LCKIELeft/1, HWA/1
  LCKIELeft/4 -> LCKLineS9/4(In4)  "<LCKLineC1>"
  LCKIELeft/2 -> LCKLineS9/2(In2)  "<LCKLineC3>"
  LCKIELeft/5 -> LCKLineS9/5(In5)  "<LCKLineC0>"
  LCKIELeft/3 -> LCKLineS9/3(In3)  "<LCKLineC2>"
  LCKIELeft/1 -> Data Type Conversion5/1  "<LCKLineValid>"
  LCKIELeft/6 -> LCKLineS9/6(In6)  "<LCKRange>"
  LCKIERight/2 -> LCKLineS10/2(In2)  "<LCKLineC3>"
  LCKIERight/5 -> LCKLineS10/5(In5)  "<LCKLineC0>"
  LCKIERight/1 -> Data Type Conversion6/1  "<LCKLineValid>"
  LCKIERight/3 -> LCKLineS10/3(In3)  "<LCKLineC2>"
  LCKIERight/4 -> LCKLineS10/4(In4)  "<LCKLineC1>"
  LCKIERight/6 -> LCKLineS10/6(In6)  "<LCKRange>"
  LCKIEOffset1/1 -> Abs2/1
  "State "/1 -> Bus Selector1/1
  Bus Selector1/1 -> Data Type Conversion/1  "<ELK_State>"
  Bus Selector1/2 -> Line/5(LKASts)  "<LKA_State>"
  Bus Selector2/1 -> [LCKSts]  "<LCK_State>"
  Bus Selector1/3 -> Line/6(LCKIESts)  "<LCKIE_State>"
  LCKSts/1 -> Bus Selector2/1
  Data Type Conversion/1 -> Line/4(ELKSts)
  Switch Case/3 -> [ELKLine]
  [ELKLine] -> LCKLineS3/Action
  [LKALine] -> LCKLineS6/Action
  [LCKIEL] -> LCKLineS9/Action
  [LCKIER] -> LCKLineS10/Action
  Compare To Constant1/1 -> Logical Operator/1
  Data Type Conversion4/1 -> LCKLineS1/1(In1)
  Data Type Conversion5/1 -> LCKLineS9/1(In1)
  Data Type Conversion6/1 -> LCKLineS10/1(In1)
  Data Type Conversion13/1 -> LCKLineS2/1(In1)
  Data Type Conversion35/1 -> Bus Creator3/1  "TarLineValid"
  LCKIEOffset/1 -> Abs3/1
  Bus Selector16/2 -> Data Type Conversion1/1  "<HWASts>"
  Data Type Conversion1/1 -> Line/2(HWAsts)
  Abs2/1 -> LCKLineS10/7(In7)
  Abs3/1 -> LCKLineS9/7(In7)
  [Select_ELKline] -> Multiport Switch1/2
  Multiport Switch1/1 -> Demux1/1
  Demux1/1 -> Bus Creator12/1  "ELK_LaneValid"
  Demux1/2 -> Bus Creator12/2  "ELK_LaneA3"
  Demux1/3 -> Bus Creator12/3  "ELK_LaneA2"
  Demux1/4 -> Bus Creator12/4  "ELK_LaneA1"
  Demux1/5 -> Bus Creator12/5  "ELK_LaneA0"
  Demux1/6 -> Bus Creator12/6  "ELK_LaneRange"
  Multiport Switch2/1 -> Demux2/1
  Demux2/1 -> Bus Creator13/1  "LKA_LaneValid"
  Demux2/2 -> Bus Creator13/2  "LKA_LaneA3"
  Demux2/3 -> Bus Creator13/3  "LKA_LaneA2"
  Demux2/4 -> Bus Creator13/4  "LKA_LaneA1"
  Demux2/5 -> Bus Creator13/5  "LKA_LaneA0"
  Demux2/6 -> Bus Creator13/6  "LKA_LaneRange"
  Bus Creator13/1 -> LKA_Lane/1
  LCK/1 -> Logical Operator/2  "<LCKLineValid>"
  Bus Creator12/1 -> ELK_Lane/1
  Logical Operator/1 -> Data Type Conversion3/1
  Data Type Conversion3/1 -> LCKLineS/1(In1)
  Line/1(y) -> Switch Case/1, [switch]
  [switch] -> Multiport Switch1/1
  Constant/1 -> Bus Creator14/1
  Constant1/1 -> Bus Creator14/3, Bus Creator14/5, Bus Creator14/6, Bus Creator14/4, Bus Creator14/2
  Bus Creator14/1 -> [default]
  [default] -> Multiport Switch1/3
  [switch] -> Multiport Switch2/1
  [default] -> Multiport Switch2/3
  LCKLineS/1(Out1) -> [LCKline]
  LCKLineS1/1(Out1) -> [TJAline]
  LCKLineS2/1(Out1) -> [HWAline]
  LCKLineS9/1(Out1) -> [IEleft]
  LCKLineS10/1(Out1) -> [IEright]
  LCKLineS3/1(Out1) -> [ELKCenterline]
  LCKLineS6/1(Out1) -> [LKAlane]
  Merge/1 -> Demux/1
  [HWAline] -> Merge/1
  [TJAline] -> Merge/2
  [ELKCenterline] -> Merge/3
  LCKLineS3/2(Out2) -> [Select_ELKline]
  "ESS_Sts "/1 -> Line/7(ESS_Sts)
  HWA2/1 -> Data Type Conversion14/1  "<ESSLineValid>"
  HWA2/2 -> ESSLine/2(In2)  "<ESSLineC3>"
  HWA2/3 -> ESSLine/3(In3)  "<ESSLineC2>"
  HWA2/4 -> ESSLine/4(In4)  "<ESSLineC1>"
  HWA2/5 -> ESSLine/5(In5)  "<ESSLineC0>"
  HWA2/6 -> ESSLine/6(In6)  "<ESSRange>"
  Switch Case/8 -> ESSLine/Action
  Data Type Conversion14/1 -> ESSLine/1(In1)
  ESSLine/1(Out1) -> [ESSline]
  Bus Selector/1 -> Data Type Conversion10/1  "<T_Valid>"
  Bus Selector/2 -> LCKLineS6/2(In2)  "<T_A3>"
  Bus Selector/3 -> LCKLineS6/3(In3)  "<T_A2>"
  Bus Selector/4 -> LCKLineS6/4(In4)  "<T_A1>"
  Bus Selector/5 -> LCKLineS6/5(In5)  "<T_A0>"
  Bus Selector/6 -> LCKLineS6/6(In6)  "<T_Range>"
  Data Type Conversion10/1 -> LCKLineS6/1(In1)
  Switch Case/7 -> LCKLineS/Action
  Demux/1 -> Data Type Conversion35/1
  LCKLineS6/2(Out2) -> [SelectLKAlane]
  [SelectLKAlane] -> Multiport Switch2/2
